simulink model "CPG_solo"  (R2015b)
settings: Solver=VariableStepAuto  StartTime=0.0  StopTime=inf  RelTol=1e-3
undefined symbols (not defined in the file or in its folder): part
settings Model: Creator=KAREN  LastModifiedBy=KAREN

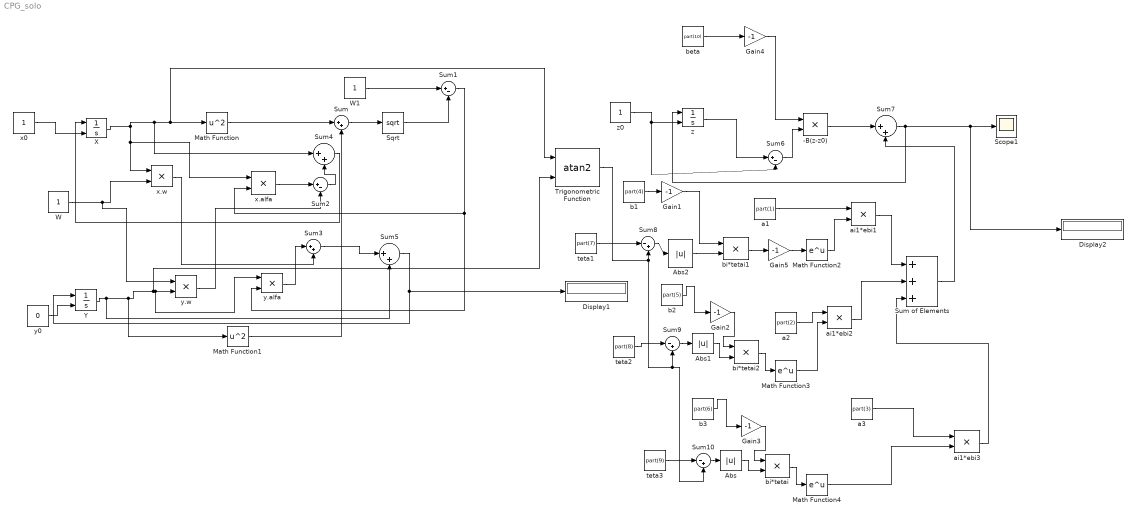
== system CPG_solo ==
  -B(z-z0) : Product
  Abs : Abs
  Abs1 : Abs
  Abs2 : Abs
  Display1 : Display
  Display2 : Display
  Gain{1..5} (5 alike) : Gain  Gain=-1
  Math Function : Math  Operator=square  SaturateOnIntegerOverflow=on
  Math Function1 : Math  Operator=square  SaturateOnIntegerOverflow=on
  Math Function2 : Math  SaturateOnIntegerOverflow=on
  Math Function3 : Math  SaturateOnIntegerOverflow=on
  Math Function4 : Math  SaturateOnIntegerOverflow=on
  Scope1 : Scope
  Sqrt : Sqrt  SaturateOnIntegerOverflow=on
  Sum{,3..5,7} (5 alike) : Sum  Inputs=|++
  Sum of Elements : Sum  Inputs=+++
  Sum1 : Sum  Inputs=|+-
  Sum10 : Sum  Inputs=|-+
  Sum2 : Sum  Inputs=|+-
  Sum6 : Sum  Inputs=|+-
  Sum8 : Sum  Inputs=|-+
  Sum9 : Sum  Inputs=|-+
  Trigonometric Function : Trigonometry  Operator=atan2
  W : Constant
  W1 : Constant
  X : Integrator  InitialConditionSource=external  InitialCondition=1
  Y : Integrator  InitialConditionSource=external
  a1 : Constant  Value=part(1)
  a2 : Constant  Value=part(2)
  a3 : Constant  Value=part(3)
  ai1*ebi1 : Product
  ai1*ebi2 : Product
  ai1*ebi3 : Product
  b1 : Constant  Value=part(4)
  b2 : Constant  Value=part(5)
  b3 : Constant  Value=part(6)
  beta : Constant  Value=part(10)
  bi*tetai : Product
  bi*tetai1 : Product
  bi*tetai2 : Product
  teta1 : Constant  Value=part(7)
  teta2 : Constant  Value=part(8)
  teta3 : Constant  Value=part(9)
  x.alfa : Product
  x.w : Product
  x0 : Constant
  y.alfa : Product
  y.w : Product
  "y0 " : Constant  Value=0
  z : Integrator  InitialConditionSource=external  InitialCondition=1
  z0 : Constant
  wires:
  Sum2/1 -> Sum4/2
  beta/1 -> Gain4/1
  Y/1 -> Sum5/2, Math Function1/1, Trigonometric Function/2, y.alfa/1, y.w/2
  Sum/1 -> Sqrt/1
  Sqrt/1 -> Sum1/2
  Math Function1/1 -> Sum/2
  bi*tetai2/1 -> Math Function3/1
  b2/1 -> Gain2/1
  Gain2/1 -> bi*tetai2/1
  teta2/1 -> Sum9/1
  a2/1 -> ai1*ebi2/1
  Trigonometric Function/1 -> Sum10/2, Sum9/2, Sum8/2
  ai1*ebi2/1 -> Sum of Elements/2
  teta3/1 -> Sum10/1
  Math Function2/1 -> ai1*ebi1/2
  b1/1 -> Gain1/1
  a1/1 -> ai1*ebi1/1
  teta1/1 -> Sum8/1
  bi*tetai1/1 -> Gain5/1
  Sum7/1 -> Display2/1, Scope1/1, z/1
  Sum5/1 -> Display1/1, Y/1
  a3/1 -> ai1*ebi3/1
  b3/1 -> Gain3/1
  -B(z-z0)/1 -> Sum7/1
  Gain3/1 -> bi*tetai/1
  bi*tetai/1 -> Math Function4/1
  X/1 -> Sum4/1, Trigonometric Function/1, Math Function/1, x.alfa/1, x.w/1
  "y0 "/1 -> Y/2
  Sum1/1 -> x.alfa/2, y.alfa/2
  z/1 -> Sum6/1
  Sum6/1 -> -B(z-z0)/2
  Math Function/1 -> Sum/1
  ai1*ebi3/1 -> Sum of Elements/3
  Sum of Elements/1 -> Sum7/2
  y.w/1 -> Sum2/2
  x.alfa/1 -> Sum2/1
  y.alfa/1 -> Sum3/1
  W1/1 -> Sum1/1
  x.w/1 -> Sum3/2
  x0/1 -> X/2
  Sum3/1 -> Sum5/1
  W/1 -> y.w/1, x.w/2
  z0/1 -> Sum6/2, z/2
  Sum10/1 -> Abs/1
  Abs/1 -> bi*tetai/2
  Sum9/1 -> Abs1/1
  Abs1/1 -> bi*tetai2/2
  Sum8/1 -> Abs2/1
  Abs2/1 -> bi*tetai1/2
  Sum4/1 -> X/1
  Gain4/1 -> -B(z-z0)/1
  Gain5/1 -> Math Function2/1
  Math Function3/1 -> ai1*ebi2/2
  Math Function4/1 -> ai1*ebi3/2
  ai1*ebi1/1 -> Sum of Elements/1
  Gain1/1 -> bi*tetai1/1
